simulink model "ground_model"  (R2023a)
settings: Solver=ode2  StartTime=0.0  StopTime=5  FixedStep=vehicle.sampletime*10  RelTol=1e-3  EnableMultiTasking=on
undefined symbols (not defined in the file or in its folder): ATOL_coeffs, defaultConsts, rwyNoise
settings Model: Creator=ac112430  LastModifiedBy=ac124458
settings SolverCC: AlgebraicLoopSolver=LineSearch
settings DataIOCC: ReturnWorkspaceOutputs=off
settings OptimizationCC: LifeSpan=inf
settings DebuggingCC: UnconnectedInputMsg=warning  UnconnectedOutputMsg=warning  UnconnectedLineMsg=warning  SFUnexpectedBacktrackingDiag=warning  SFNoUnconditionalDefaultTransitionDiag=warning  SFExecutionAtInitializationDiag=none  ArithmeticOperatorsInVariantConditions=warning
settings ModelReferenceCC: EnableRefExpFcnMdlSchedulingChecks=on
settings SFSimCC: SimUseLocalCustomCode=off  CustomCodeUndefinedFunction=UseInterfaceOnly
settings RTWCC: RTWUseLocalCustomCode=off
settings CodeAppCC: StateflowObjectComments=on
settings GRTTargetCC: TargetLangStandard=C89/C90 (ANSI)
settings ConfigComp: CovMetricSettings=dw  CovSaveCumulativeToWorkspaceVar=on  CovSaveSingleToWorkspaceVar=on  CovExternalEMLEnable=off

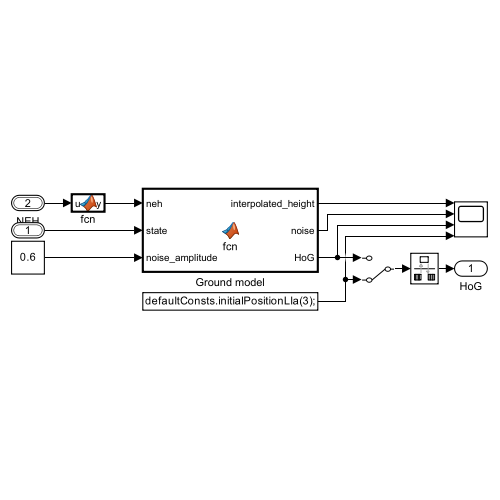
[thumbnail: Simulink's stored preview of the top-level diagram]
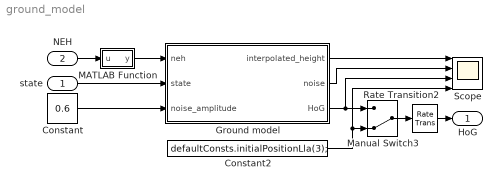
== system ground_model ==
  state : Inport  OutDataTypeStr=Bus: fmBus
  NEH : Inport  Port=2  OutDataTypeStr=Bus: rnwy_monitor
  Constant : Constant  Value=0.6
  Constant2 : Constant  Value=defaultConsts.initialPositionLla(3);
  Ground model : MATLAB Function  TreatAsAtomicUnit=on
  MATLAB Function : MATLAB Function  TreatAsAtomicUnit=on
  Manual Switch3 : ManualSwitch  CurrentSetting=0
  Rate Transition2 : RateTransition
  Scope : Scope  NumInputPorts=4
  HoG : Outport
  wires:
  state/1 -> Ground model/2(state)
  Manual Switch3/1 -> Rate Transition2/1
  Ground model/2(noise) -> Scope/2
  Constant2/1 -> Manual Switch3/2, Scope/4
  Ground model/3(HoG) -> Manual Switch3/1, Scope/3
  Ground model/1(interpolated_height) -> Scope/1
  Constant/1 -> Ground model/3(noise_amplitude)
  MATLAB Function/1(y) -> Ground model/1(neh)
  NEH/1 -> MATLAB Function/1(u)
  Rate Transition2/1 -> HoG/1

== matlab function ground_model/MATLAB Function ==
  data: u input Bus: rnwy_monitor; y output single size=[3 6]
function y = fcn(u)

y = single([u.north';u.east';u.altitude']);

== matlab function ground_model/Ground model ==
  data: interpolated_height output; noise output; neh input single size=[3 6]; state input; HoG output; ATOL_coeffs parameter; rwyNoise parameter; noise_amplitude input
function [interpolated_height, noise, HoG] = fcn(neh, state, ATOL_coeffs, rwyNoise, noise_amplitude)

% get params
TOLen = ATOL_coeffs(1);
TOHdg = ATOL_coeffs(2)*pi/180;
TODeltaAlt = (ATOL_coeffs(5) - ATOL_coeffs(24))*10^-3;
LDGLen = ATOL_coeffs(6);
LDGHdg = ATOL_coeffs(7)*pi/180;
LDGDeltaAlt = (ATOL_coeffs(10) - ATOL_coeffs(25))*10^-3;
pos = state.rigidbodyBus.xg;

% get runway points
P1 = neh(:,1);                                                      %TO start
P2 = P1 + [TOLen*cos(TOHdg), TOLen*sin(TOHdg), TODeltaAlt]';        %TO end
P3 = neh(:,5);                                                      %LDG start
P4 = P3 + [LDGLen*cos(LDGHdg), LDGLen*sin(LDGHdg), LDGDeltaAlt]';   %TO end
approach_fix = neh(:,4);

% interpolate between runway points
interpolated_height = interpolate_all([P1, P2, P3, P4], pos);

% calculate noise map offset
min_pts = min([P1,P2,P3,P4,approach_fix],[],2);
max_pts = max([P1,P2,P3,P4,approach_fix],[],2);
center_pts = max_pts(1:2)/2 + min_pts(1:2)/2;
center_map = size(rwyNoise)'/2;
offset = center_map - center_pts;

% find position wrt. noise plot
pos_noise = pos(1:2) + offset;
%noise = interp2(0:(size(rwyNoise,1)-1),0:(size(rwyNoise,2)-1),rwyNoise',pos_noise(1),pos_noise(2),'linear',0);
if any(pos_noise < 1) || any(pos_noise > size(rwyNoise)')
    noise = 0;
else
    A = rwyNoise(floor(pos_noise(1)), floor(pos_noise(2)));
    B = rwyNoise(ceil(pos_noise(1)), floor(pos_noise(2)));
    C = rwyNoise(floor(pos_noise(1)), ceil(pos_noise(2)));
    D = rwyNoise(ceil(pos_noise(1)), ceil(pos_noise(2)));
    delta = pos_noise-floor(pos_noise);
    noise = noise_amplitude*double((1-delta(1))*(1-delta(2))*A + delta(1)*(1-delta(2))*B + delta(2)*(1-delta(1))*C + delta(1)*delta(2)*D);
end

% add noise
HoG = double(interpolated_height + noise);
end

function interpolated_height = interpolate_all(points, pos)

    diff = [points(:,1)-points(:,3), points(:,1)-points(:,4), points(:,2)-points(:,3), points(:,2)-points(:,4)];
    compare = vecnorm(diff(1:2,:));

    i=1*all(compare(1:2));
    j=2*all(compare(3:4));

    pts_use = [points(:,1:i), points(:,2:j), points(:,3:4)];

    if size(pts_use,2) == 2
        % two surface points
        g12 = pts_use(:,2)-pts_use(:,1);
        g1p = pos - pts_use(:,1);
        dist = dot(g12(1:2), g1p(1:2))/dot(g12(1:2), g12(1:2));
        interpolated_height = -(pts_use(3,1)+dist*g12(3));
    elseif size(pts_use,2) == 3
        % three surface points
        interpolated_height = -interpolate_triangle(pts_use, pos);
    elseif size(pts_use,2) == 4
        % four surface points   
        % check if one point is on the inside
        [inside1, frame1] = check_inside(pts_use(1:2,[2,3,4]), pts_use(1:2,1),2,3,4);
        [inside2, frame2] = check_inside(pts_use(1:2,[1,3,4]), pts_use(1:2,2),1,3,4);
        [inside3, frame3] = check_inside(pts_use(1:2,[1,2,4]), pts_use(1:2,3),1,2,4);
        [inside4, frame4] = check_inside(pts_use(1:2,[1,2,3]), pts_use(1:2,4),1,2,3);
        inside = [inside1, inside2, inside3, inside4];
        frame = [frame1, frame2, frame3, frame4];

        if any(inside)
            % 3 planes
            [~,i]=max(inside);
            j = [1:i-1,i+1:4];
            sectors = [atan2(pts_use(2,j(1))-pts_use(2,i), pts_use(1,j(1))-pts_use(1,i)), ...
                       atan2(pts_use(2,j(2))-pts_use(2,i), pts_use(1,j(2))-pts_use(1,i)), ...
                       atan2(pts_use(2,j(3))-pts_use(2,i), pts_use(1,j(3))-pts_use(1,i))];
            [~,order] = sort(sectors);

            position_line = atan2(pos(2)-pts_use(2,i), pos(1)-pts_use(1,i));
            if position_line >= sectors(order(1)) && position_line <= sectors(order(2)) % in first sector
                interpolated_height = -interpolate_triangle(pts_use(:,[i, j(order(1)), j(order(2))]), pos);  
            elseif position_line >= sectors(order(2)) && position_line <= sectors(order(3)) % in second sector
                interpolated_height = -interpolate_triangle(pts_use(:,[i, j(order(2)), j(order(3))]), pos);  
            else % in other sector
                interpolated_height = -interpolate_triangle(pts_use(:,[i, j(order(3)), j(order(1))]), pos);  
            end
        elseif any(frame)
            % one point lies on another runway - find point
            [pt,i]=max(frame);
            % dividing line is pt-i
            % common line: pt-i
            if pt<i
                sector_points = [pt, i];
            else
                sector_points = [i, pt];
            end
            close_points = [1:pt-1, pt+1:i-1,i+1:4];
            dist=vecnorm(pts_use(1:2,close_points)-pos(1:2));
            [~,i] = min(dist);
            closest = close_points(i);
            interpolated_height = -interpolate_triangle(pts_use(:,[sector_points(1),sector_points(2),closest]), pos);   
        else
            % point cloud is convex, 
            % check if runways 12 and 34 are parallel
            s12 = pts_use(1:2,2)-pts_use(1:2,1);
            s34 = pts_use(1:2,4)-pts_use(1:2,3);
            rwy_parallel = norm(s12)*norm(s34)==dot(s12,s34);

            % check if runways intersect
            rwy_intersect = 0;
            if ~rwy_parallel % runways not parallel
                rwy_intersect = intersect_lines(pts_use(1:2,1:2),pts_use(1:2,3:4));
            end

            if rwy_intersect
                % make TO runwy sloped and LDG runway flat
                % planes 134 and 234, common line: 34
                % check sector
                close_points = [1, 2];
                dist=vecnorm(pts_use(1:2,close_points)-pos(1:2)*ones(1,2));
                [~,i] = min(dist);
                closest = close_points(i);
                interpolated_height = -interpolate_triangle(pts_use(:,[3,4,closest]), pos);
            else 
            %runways do not intersect
                % find out if 31 intersects with 41 or 42
                intersect_13_14 = intersect_lines(pts_use(1:2,[1,3]),pts_use(1:2,[1,4]));
                intersect_13_24 = intersect_lines(pts_use(1:2,[1,3]),pts_use(1:2,[2,4]));

                if intersect_13_14 || intersect_13_24
                    % planes 234, 124, common line: 24
                    % check sector
                    close_points = [1, 3];
                    dist=vecnorm(pts_use(1:2,close_points)-pos(1:2)*ones(1,2));
                    [~,i] = min(dist);
                    closest = close_points(i);
                    interpolated_height = -interpolate_triangle(pts_use(:,[2,4,closest]), pos);
                else
                    %planes 134, 124, common line: 14
                    % check sector
                    close_points = [2, 3];
                    dist=vecnorm(pts_use(1:2,close_points)-pos(1:2)*ones(1,2));
                    [~,i] = min(dist);
                    closest = close_points(i);
                    interpolated_height = -interpolate_triangle(pts_use(:,[1,4,closest]), pos);
                end
            end
        end
    else
        interpolated_height = single(0);
    end
end

function HoG = interpolate_triangle(pos_matrix, pos)
    % interpolate ground altitude (Barycentric Coordinates)
    den = (pos_matrix(2,2)-pos_matrix(2,3))*(pos_matrix(1,1)-pos_matrix(1,3))+(pos_matrix(1,3)-pos_matrix(1,2))*(pos_matrix(2,1)-pos_matrix(2,3));
    weight1 = ((pos_matrix(2,2)-pos_matrix(2,3))*(pos(1)-pos_matrix(1,3))+(pos_matrix(1,3)-pos_matrix(1,2))*(pos(2)-pos_matrix(2,3)))/den;
    weight2 = ((pos_matrix(2,3)-pos_matrix(2,1))*(pos(1)-pos_matrix(1,3))+(pos_matrix(1,1)-pos_matrix(1,3))*(pos(2)-pos_matrix(2,3)))/den;
    weight3 = 1-weight1-weight2;
    HoG = weight1*pos_matrix(3,1)+weight2*pos_matrix(3,2)+weight3*pos_matrix(3,3);
end

function [inside, frame] = check_inside(triangle,probe,w1,w2,w3)
    v  = probe;
    v0 = triangle(:,1);
    v1 = triangle(:,2)-triangle(:,1);
    v2 = triangle(:,3)-triangle(:,1);
    a = (det([v,v2])-det([v0,v2]))/det([v1,v2]);
    b = (det([v,v1])-det([v0,v1]))/det([v1,v2]);
    
    inside = a>0 && b<0 && a+b<1;
    frame = w2*(a==0 && b<0 && b>-1) + w3*(b==0 && a>0 && a<1) + w1*(a+b==0 && a>0 && a<1 && b<0 && b>-1);
    % if a == 0 or b == 0 or a+b == 0: point on other line
    % if a>0 and b>0 and a+b<1
end

function rwy_intersect = intersect_lines(p12,p34)
            % TO rwy:  g = p1+s*(p2-p1)
            % LDG rwy: h = p3+t*(p4-p3)
            % p1-p3 + s*(p2-p1) = t*(p4-p3)
    p1x = p12(1,1);
    p2x = p12(1,2);
    p1y = p12(2,1);
    p2y = p12(2,2);
    p3x = p34(1,1);
    p4x = p34(1,2);
    p3y = p34(2,1);
    p4y = p34(2,2);
    t = ((p1x-p3x)*(p2y-p1y)-(p1y-p3y)*(p2x-p1x))/((p4x-p3x)*(p2y-p1y)-(p4y-p3y)*(p2x-p1x));
    s = ((p1x-p3x)*(p4y-p3y)-(p1y-p3y)*(p4x-p3x))/((p4x-p3x)*(p2y-p1y)-(p4y-p3y)*(p2x-p1x));
    if isinf(s) || isinf(t)
        rwy_intersect = 0;
    else
        rwy_intersect = double(t>0 && t<1 && s>0 && s<1);
    end
end
